simulink model "Regularization"  (Simulink 7.6)
settings: Solver=FixedStepDiscrete  StartTime=0.0  StopTime=60*60*4  FixedStep=300  RelTol=1e-3
values from neighbouring files (symbols this model uses):
  A_ahuflow = [1 0]    [RegularizationData.mat]
  A_DATtoZones = [1 0 0 0 0 0 0 0 0 0 0 0 ... (648 elements, 18x36)]    [RegularizationData.mat]
  A_fan_sup = [3 2 1 0]    [RegularizationData.mat]
  A_mapMatrixVAV2Zones1 = [1 0 0 0 0 0 0 0 0 0 0 0 ... (324 elements, 18x18)]    [RegularizationData.mat]
  A_mdots_boundsMax = [1 0 0 0 0 0 0 0 0 0 0 0 ... (1296 elements, 36x36)]    [RegularizationData.mat]
  A_mdots_boundsMin = [1 0 0 0 0 0 0 0 0 0 0 0 ... (1296 elements, 36x36)]    [RegularizationData.mat]
  A_OADtoOAF = [2 1 0]    [RegularizationData.mat]
  A_ObjFun = [1 0 0 0 0 1 0 0 0 0 1 0 ... (20 elements, 4x5)]    [RegularizationData.mat]
  A_returnT1 = [1 0 0 0 0 0 0 0 0 0 0 0 ... (324 elements, 18x18)]    [RegularizationData.mat]
  A_sum_DAT = [1 0 0 0 0 0 0 0 0 0 0 0 ... (361 elements, 19x19)]    [RegularizationData.mat]
  A_sumMdots1 = [1 0 0 0 0 0 0 0 0 0 0 0 ... (324 elements, 18x18)]    [RegularizationData.mat]
  A_Tzone_bounds1 = [1 0 0 0 0 0 0 0 0 0 0 0 ... (729 elements, 27x27)]    [RegularizationData.mat]
  A_VAV_DAT = [1 1 1 1 1 1 1 1 1 1 1 1 ... (666 elements, 18x37)]    [RegularizationData.mat]
  A_VAV_Energy = [0 1 0 1 0 1 0 1 0 1 0 1 ... (1332 elements, 36x37)]    [RegularizationData.mat]
  A_vlvcomd_boundsMax = [1 0 0 0 0 0 0 0 0 0 0 0 ... (1296 elements, 36x36)]    [RegularizationData.mat]
  A_vlvcomd_boundsMin = [1 0 0 0 0 0 0 0 0 0 0 0 ... (1296 elements, 36x36)]    [RegularizationData.mat]
  Azone =     [RegularizationData.mat]
  C_ahuflow = [0.90501 7.4491]    [RegularizationData.mat]
  C_DATtoZones = [1 0 0 0 0 0 0 0 0 1 0 0 ... (162 elements, 9x18)]    [RegularizationData.mat]
  C_fan_sup = [0.007418 -0.1732 2.207 -5.847]    [RegularizationData.mat]
  C_mapMatrixVAV2Zones1 = [1 0 0 0 0 0 0 0 0 0.813953488 0 0 ... (162 elements, 9x18)]    [RegularizationData.mat]
  C_mdots_boundsMax = [1 0 0 0 0 0 0 0 0 0 0 0 ... (648 elements, 18x36)]    [RegularizationData.mat]
  C_mdots_boundsMin = [1 0 0 0 0 0 0 0 0 0 0 0 ... (648 elements, 18x36)]    [RegularizationData.mat]
  C_OADtoOAF = [-2.3694 4.3066 -1.008]    [RegularizationData.mat]
  C_ObjFun = [3 1 1 1]    [RegularizationData.mat]
  C_returnT1 = [1 1 1 1 1 1 1 1 1 -0.4 -0.4 -0.4 ... (18 elements, 1x18)]    [RegularizationData.mat]
  C_sum_DAT = [1 1 1 1 1 1 1 1 1 1 1 1 ... (342 elements, 18x19)]    [RegularizationData.mat]
  C_sumMdots1 = [1 1 1 1 1 1 1 1 1 1 1 1 ... (18 elements, 1x18)]    [RegularizationData.mat]
  C_Tzone_boundsMax1 = [1 0 0 0 0 0 0 0 0 0 1 0 ... (243 elements, 9x27)]    [RegularizationData.mat]
  C_Tzone_boundsMin1 = [1 0 0 0 0 0 0 0 0 0 1 0 ... (243 elements, 9x27)]    [RegularizationData.mat]
  C_VAV_DAT = [0.253505482147 0 0 0 0 0 0 0 0 0 0 0 ... (324 elements, 18x18)]    [RegularizationData.mat]
  C_VAV_Energy = [1 0 0 0 0 0 0 0 0 0 0 0 ... (648 elements, 18x36)]    [RegularizationData.mat]
  C_vlvcomd_boundsMax = [1 0 0 0 0 0 0 0 0 0 0 0 ... (648 elements, 18x36)]    [RegularizationData.mat]
  C_vlvcomd_boundsMin = [1 0 0 0 0 0 0 0 0 0 0 0 ... (648 elements, 18x36)]    [RegularizationData.mat]
  cp_air = 1.006    [RegularizationData.mat]
  cp_w = 4.18    [RegularizationData.mat]
  Czone =     [RegularizationData.mat]
  d = [0.040172538 0.168105054 0.715382539]    [RegularizationData.mat]
  DAT_init = 18.3333333333    [RegularizationData.mat]
  DAT_max_init = 24.4444444444    [RegularizationData.mat]
  DAT_min_init = 12.7777777778    [RegularizationData.mat]
  DAT_step_cost = 5    [RegularizationData.mat]
  dTfan_const = 1    [RegularizationData.mat]
  eff_hc_max = 0.7    [RegularizationData.mat]
  HWST_init = 48.8888888889    [RegularizationData.mat]
  MaxAirFlow1 = 22.6524    [RegularizationData.mat]
  MaxZoneT = [26 26 26 26 26 26 26 26 26]    [RegularizationData.mat]
  mdotsa_init = [0.25 0.25 0.25 0.25 0.25 0.25 0.25 0.25 0.25 0.25 0.25 0.25 ... (18 elements, 18x1)]    [RegularizationData.mat]
  mdotsa_vav_max = [2 2 2 2 2 2 2 2 2 2 2 2 ... (18 elements, 18x1)]    [RegularizationData.mat]
  mdotsa_vav_min = [0.2 0.2 0.2 0.2 0.2 0.2 0.2 0.2 0.2 0.2 0.2 0.2 ... (18 elements, 18x1)]    [RegularizationData.mat]
  mdotw_max = 5.868    [RegularizationData.mat]
  MinAirFlow1 = 2.03881295462    [RegularizationData.mat]
  MinZoneT = [19 19 19 19 19 19 19 19 19]    [RegularizationData.mat]
  NumVAV1 = 18    [RegularizationData.mat]
  NumZones1 = 9    [RegularizationData.mat]
  OAD_high = 1    [RegularizationData.mat]
  OAD_init = 0.5    [RegularizationData.mat]
  OAD_low = 0.3    [RegularizationData.mat]
  params =     [RegularizationData.mat]
  SlackVariable_Weight = 10000    [RegularizationData.mat]
  vlvcomd_init = [0.01 0.01 0.01 0.01 0.01 0.01 0.01 0.01 0.01 0.01 0.01 0.01 ... (18 elements, 1x18)]    [RegularizationData.mat]
  vlvcomd_vav_high = [1 1 1 1 1 1 1 1 1 1 1 1 ... (18 elements, 18x1)]    [RegularizationData.mat]
  vlvcomd_vav_low = [0.002 0.002 0.002 0.002 0.002 0.002 0.002 0.002 0.002 0.002 0.002 0.002 ... (18 elements, 18x1)]    [RegularizationData.mat]
  vlvComdMin = [0.001 0.001 0.001 0.001 0.001 0.001 0.001 0.001 0.001 0.001 0.001 0.001 ... (18 elements, 18x1)]    [RegularizationData.mat]
undefined symbols (not defined in the file or in its folder): DAT, DAT_min, DAT_min_ext, dTfan, MAT, mdot_a, mdotsa, mdotsa_SP, OAD, prevDAT, slack, slack_weight, sparse, T, Thd, Thws, TLB, Tmix, TUB, Twin, vav_energy, vlv, vlv_comd, x1, x2
libraries: MPCMdlLib x75
settings Model: Creator=trckam  LastModifiedBy=sergv

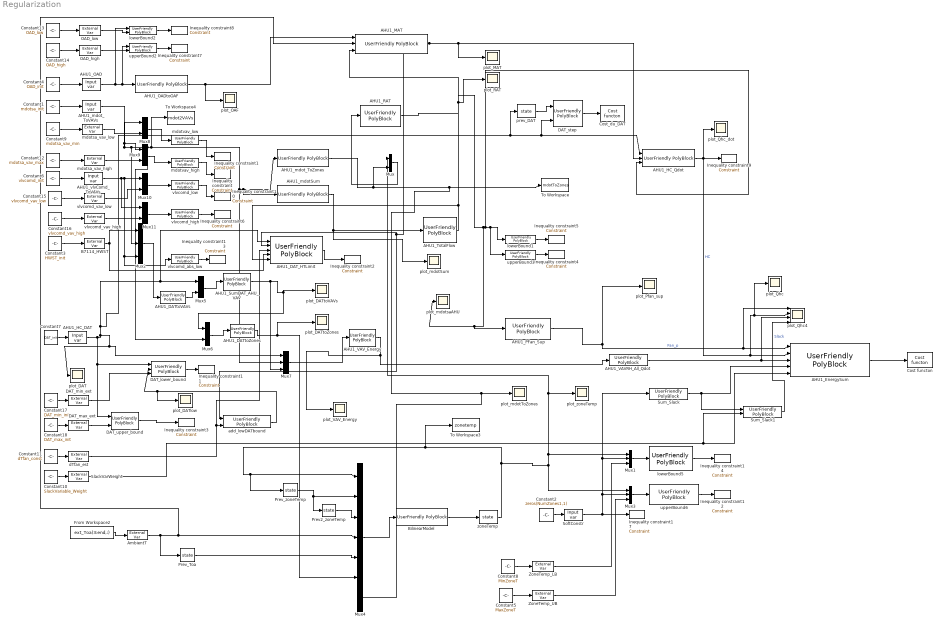
== system Regularization ==
  AHU1_DAT_HTLimit : MPCMdlLib/UserFriendly PolyBlock  Tag=PolyBlock  A=[1 0 0 0 1;0 1 0 0 1;0 0 1 0 1;0 1 0 0 0;0 0 0 1 0]  C=[cp_air, -cp_air, -cp_air, +eff_hc_max*mdotw_max*cp_w, -eff_hc_max*mdotw_max*cp_w]  gA=[0 0 0 0 0]  gC=[1]  input_type=Scalar  output_type=Scalar  port_names=DAT,MAT,dTfan,Twin,mdotsa
  AHU1_DATtoVAVs : MPCMdlLib/UserFriendly PolyBlock  Tag=PolyBlock  A=A_VAV_DAT  C=C_VAV_DAT  gA=zeros(1,37)  gC=[1]  input_type=Vector  output_type=Vector  port_names=Thws,mdotsa_SP[1-18],vlv_comd[1-18]
  AHU1_DATtoZones : MPCMdlLib/UserFriendly PolyBlock  Tag=PolyBlock  A=A_DATtoZones  C=C_DATtoZones  gA=Ag_DATtoZones  gC=Cg_DATtoZones  input_type=Vector  output_type=Vector  port_names=x1,x2
  AHU1_EnergySum : MPCMdlLib/UserFriendly PolyBlock  Tag=PolyBlock  A=A_ObjFun  C=C_ObjFun  gA=zeros(1,size(A_ObjFun,2))  gC=1  input_type=Scalar  output_type=Scalar  port_names=Pfan, Qhc, Qrh,slack,slack_weight
  AHU1_HC_DAT : MPCMdlLib/Input var  Tag=OptInput  SystemSampleTime=-1  step_ratio=1  save_name=BL_AHU1_HC_DAT
  AHU1_HC_Qdot : MPCMdlLib/UserFriendly PolyBlock  Tag=PolyBlock  A=[1 0 1;0 1 1;0 0 1]  C=[cp_air, -cp_air, -cp_air]  gA=[0 0 0]  gC=[1]  input_type=Scalar  output_type=Scalar  port_names=Thd,Tmix,mdot_a
  AHU1_MAT : MPCMdlLib/UserFriendly PolyBlock  Tag=PolyBlock  A=[1 1 0; 0 0 1;1 0 1]  C=[1 1 -1]  gA=[0 0 0]  gC=1  input_type=Scalar  output_type=Scalar  port_names=frac,amb, ret
  AHU1_OAD : MPCMdlLib/Input var  Tag=OptInput  SystemSampleTime=-1  step_ratio=1  save_name=BL_AHU1_OAD
  AHU1_OADtoOAF : MPCMdlLib/UserFriendly PolyBlock  Tag=PolyBlock  A=A_OADtoOAF  C=C_OADtoOAF  gA=[0]  gC=1  input_type=Scalar  output_type=Scalar  port_names=OAD
  AHU1_PFan_Sup : MPCMdlLib/UserFriendly PolyBlock  Tag=PolyBlock  A=A_fan_sup  C=C_fan_sup  gA=[0 ]  gC=1  input_type=Scalar  output_type=Scalar  port_names=mdot_a
  AHU1_RAT : MPCMdlLib/UserFriendly PolyBlock  Tag=PolyBlock  A=A_returnT1  C=C_returnT1  gA=gA_returnT1  gC=Cg_returnT1  input_type=Vector  output_type=Scalar  port_names=x1,x2
  AHU1_SumDAT_AHU_VAV : MPCMdlLib/UserFriendly PolyBlock  Tag=PolyBlock  A=A_sum_DAT  C=C_sum_DAT  gA=zeros(1,19)  gC=1  input_type=Vector  output_type=Vector  port_names=x1,x2
  AHU1_TotalFlow : MPCMdlLib/UserFriendly PolyBlock  Tag=PolyBlock  A=A_ahuflow  C=C_ahuflow  gA=[ 0]  gC=1  input_type=Scalar  output_type=Scalar  port_names=mdotvav
  AHU1_VAVRH_All_Qdot : MPCMdlLib/UserFriendly PolyBlock  Tag=PolyBlock  A=eye(NumVAV1)  C=ones(1,NumVAV1)  gA=zeros(1,NumVAV1)  gC=1  input_type=Vector  output_type=Scalar  port_names=vav_energy[1-9]
  AHU1_VAV_Energy : MPCMdlLib/UserFriendly PolyBlock  Tag=PolyBlock  A=A_VAV_Energy  C=C_VAV_Energy  gA=zeros(1,37)  gC=1  input_type=Vector  output_type=Vector  port_names=x1,x2
  AHU1_mdotSum : MPCMdlLib/UserFriendly PolyBlock  Tag=PolyBlock  A=A_sumMdots1  C=C_sumMdots1  gA=sparse(1,size(A_sumMdots1,2),0)  gC=1  input_type=Vector  output_type=Vector  port_names=x1,x2
  AHU1_mdot_ToVAVs : MPCMdlLib/Input var  Tag=OptInput  SystemSampleTime=-1  step_ratio=1  save_name=BL_AHU1_mdot_ToVAVs
  AHU1_mdot_ToZones : MPCMdlLib/UserFriendly PolyBlock  Tag=PolyBlock  A=A_mapMatrixVAV2Zones1  C=C_mapMatrixVAV2Zones1  gA=sparse(1,size(A_mapMatrixVAV2Zones1,2),0)  gC=1  input_type=Vector  output_type=Vector  port_names=x1,x2
  AHU1_vlvComd_ToVAVs : MPCMdlLib/Input var  Tag=OptInput  SystemSampleTime=-1  step_ratio=1  save_name=BL_AHU1_vlvComd_ToVAVs
  AmbientT : MPCMdlLib/External Var  Tag=OptExternal  SystemSampleTime=-1  save_name=BL_AmbientT
  B7114_HWST : MPCMdlLib/External Var  Tag=OptExternal  SystemSampleTime=-1  save_name=BL_B7114_HWST
  BilinearModel : MPCMdlLib/UserFriendly PolyBlock  Tag=PolyBlock  A=Azone  C=Czone  gA=sparse(1,size(Azone,2),0)  gC=1  input_type=Vector  output_type=Vector  port_names=UU
  Constant1 : Constant  Value=mdotsa_init
  Constant10 : Constant  Value=SlackVariable_Weight
  Constant11 : Constant  Value=dTfan_const
  Constant12 : Constant  Value=mdotsa_vav_max
  Constant13 : Constant  Value=OAD_low
  Constant14 : Constant  Value=OAD_high
  Constant15 : Constant  Value=vlvcomd_vav_low
  Constant16 : Constant  Value=vlvcomd_vav_high
  Constant17 : Constant  Value=DAT_min_init
  Constant18 : Constant  Value=DAT_max_init
  Constant2 : Constant  Value=zeros(NumZones1,1)
  Constant3 : Constant  Value=HWST_init
  Constant4 : Constant  Value=OAD_init
  Constant5 : Constant  Value=MaxZoneT
  Constant6 : Constant  Value=vlvcomd_init
  Constant7 : Constant  Value=DAT_init
  Constant8 : Constant  Value=MinZoneT
  Constant9 : Constant  Value=mdotsa_vav_min
  Cost functon : MPCMdlLib/Cost functon  Tag=OptCost
  "Cost_du_DAT " : MPCMdlLib/Cost functon  Tag=OptCost
  DAT_lower_bound : MPCMdlLib/UserFriendly PolyBlock  Tag=PolyBlock  A=[1 0 0;0 1 0;0 0 1]  C=[1 -1 0;1 0 -1]  gA=[0 0 0]  gC=1  input_type=Scalar  output_type=Vector  port_names=DAT,DAT_min,DAT_min_ext
  DAT_max_ext : MPCMdlLib/External Var  Tag=OptExternal  SystemSampleTime=-1  save_name=BL_DAT_max_ext
  DAT_min_ext : MPCMdlLib/External Var  Tag=OptExternal  SystemSampleTime=-1  save_name=BL_DAT_min_ext
  DAT_step : MPCMdlLib/UserFriendly PolyBlock  Tag=PolyBlock  A=[2 0 ; 1 1 ; 0 2]  C=[1 -2 1]*DAT_step_cost  gA=[0 0]  gC=1  input_type=Scalar  output_type=Scalar  port_names=DAT,prevDAT
  DAT_upper_bound : MPCMdlLib/UserFriendly PolyBlock  Tag=PolyBlock  A=[1 0;0 1]  C=[1 -1]  gA=[0 0]  gC=1  input_type=Scalar  output_type=Scalar  port_names=DAT, DAT_max
  From Workspace2 : FromWorkspace  VariableName=ext_Toa(3:end,:)  SampleTime=300
  Inequality constraint{,2..4,6..7,12} (7 alike) : MPCMdlLib/Constraint  Tag=InequalBlock  CompareSign=< 0
  Inequality constraint{1,5,8..11,13..14,17} (9 alike) : MPCMdlLib/Constraint  Tag=InequalBlock  CompareSign=> 0
  Mux{,5..6,8..11} (7 alike) : Mux  Inputs=2
  Mux{1..3,7} (4 alike) : Mux  Inputs=3
  Mux4 : Mux  Inputs=7
  OAD_high : MPCMdlLib/External Var  Tag=OptExternal  SystemSampleTime=-1  save_name=BL_OAD_high
  OAD_low : MPCMdlLib/External Var  Tag=OptExternal  SystemSampleTime=-1  save_name=BL_OAD_low
  Prev2_zoneTemp : MPCMdlLib/state  Tag=OptState  SystemSampleTime=-1  init_val=params.y0(1,:)  save_name=BL_Prev2_zoneTemp
  Prev_Toa : MPCMdlLib/state  Tag=OptState  SystemSampleTime=-1  init_val=ext_Toa(2,2:end)  save_name=BL_Prev_Toa
  Prev_zoneTemp : MPCMdlLib/state  Tag=OptState  SystemSampleTime=-1  init_val=params.y0(2,:)  save_name=BL_Prev_zoneTemp
  SlackVarWeight : MPCMdlLib/External Var  Tag=OptExternal  SystemSampleTime=-1  save_name=BL_SlackVarWeight
  SoftConstr : MPCMdlLib/Input var  Tag=OptInput  SystemSampleTime=-1  step_ratio=1  save_name=BL_SoftConstr
  Sum_Slack : MPCMdlLib/UserFriendly PolyBlock  Tag=PolyBlock  A=eye(NumZones1)  C=ones(1,NumZones1)  gA=zeros(1,NumZones1)  gC=1  input_type=Vector  output_type=Scalar  port_names=slack[1-1000]
  Sum_Slack1 : MPCMdlLib/UserFriendly PolyBlock  Tag=PolyBlock  A=[1 1]  C=[1]  gA=[0 0]  gC=1  input_type=Scalar  output_type=Scalar  port_names=slack,slack_weight
  To Workspace : ToWorkspace  VariableName=mdotToZones  SampleTime=-1  SaveFormat=Structure
  To Workspace3 : ToWorkspace  VariableName=zonetemp  SampleTime=-1  SaveFormat=Structure
  To Workspace4 : ToWorkspace  VariableName=mdot2VAVs  SampleTime=-1  SaveFormat=Structure
  ZoneTemp_LB : MPCMdlLib/External Var  Tag=OptExternal  SystemSampleTime=-1  save_name=BL_ZoneTemp_LB
  ZoneTemp_UB : MPCMdlLib/External Var  Tag=OptExternal  SystemSampleTime=-1  save_name=BL_ZoneTemp_UB
  add_lowDATbound : MPCMdlLib/UserFriendly PolyBlock  Tag=PolyBlock  A=[1 0;0 1]  C=[1 1]  gA=[0 0]  gC=1  input_type=Scalar  output_type=Scalar  port_names=MAT,dTfan
  dTfan_est : MPCMdlLib/External Var  Tag=OptExternal  SystemSampleTime=-1  save_name=BL_dTfan_est
  lowerBound1 : MPCMdlLib/UserFriendly PolyBlock  Tag=PolyBlock  A=[1; 0]  C=[1 -MinAirFlow1]  gA=[0 ]  gC=1  input_type=Scalar  output_type=Scalar  port_names=x1
  lowerBound2 : MPCMdlLib/UserFriendly PolyBlock  Tag=PolyBlock  A=[1 0;0 1]  C=[1 -1]  gA=[0 0]  gC=1  input_type=Scalar  output_type=Scalar  port_names=OAD, OAD_low
  lowerBound5 : MPCMdlLib/UserFriendly PolyBlock  Tag=PolyBlock  A=A_Tzone_bounds1  C=C_Tzone_boundsMin1  gA=sparse(1,size(A_Tzone_bounds1,2),0)  gC=1  input_type=Vector  output_type=Vector  port_names=T[1-9],d[1-9],TLB[1-9]
  mdotsa_vav_high : MPCMdlLib/External Var  Tag=OptExternal  SystemSampleTime=-1  save_name=BL_mdotsa_vav_high
  mdotsa_vav_low : MPCMdlLib/External Var  Tag=OptExternal  SystemSampleTime=-1  save_name=BL_mdotsa_vav_low
  mdotvav_high : MPCMdlLib/UserFriendly PolyBlock  Tag=PolyBlock  A=A_mdots_boundsMax  C=C_mdots_boundsMax  gA=sparse(1,size(A_mdots_boundsMax,2),0)  gC=1  input_type=Vector  output_type=Vector  port_names=x1,x2
  mdotvav_low : MPCMdlLib/UserFriendly PolyBlock  Tag=PolyBlock  A=A_mdots_boundsMin  C=C_mdots_boundsMin  gA=sparse(1,size(A_mdots_boundsMin,2),0)  gC=1  input_type=Vector  output_type=Vector  port_names=x1,x2
  plot_DAT : Scope
      settings: TimeRange=6000  YMin=21.30200235571261  YMax=22.1020023557126  SaveName=ScopeData11
  plot_DATlow : Scope
      settings: TimeRange=6000  YMin=21.30200235571261  YMax=22.1020023557126  SaveName=ScopeData12
  plot_DATtoVAVs : Scope
      settings: TimeRange=6000  YMin=21.30200235571261  YMax=22.1020023557126
  plot_DATtoZones : Scope
      settings: TimeRange=6000  YMin=21.30200235571261  YMax=22.1020023557126  SaveName=ScopeData3
  plot_MAT : Scope
      settings: TimeRange=15000  YMin=20  YMax=25  SaveName=ScopeData10
  plot_OAF : Scope
      settings: TimeRange=14400  YMin=21.25  YMax=24.5  SaveName=ScopeData7
  plot_Pfan_sup : Scope
      settings: TimeRange=14400  YMin=21.25  YMax=24.5  SaveName=ScopeData2
  plot_Qhc : Scope
      settings: TimeRange=14400  YMin=21.25  YMax=24.5  SaveName=ScopeData13
  plot_Qhc4 : Scope  NumInputPorts=4
      settings: TimeRange=14400  YMin=21.25~-5~-5~-5  YMax=24.5~5~5~5  SaveName=ScopeData17
  plot_Qhc_dot : Scope
      settings: TimeRange=15000  YMin=89  YMax=96  SaveName=ScopeData6
  plot_RAT : Scope
      settings: TimeRange=14400  YMin=9.236459999999999  YMax=10.2087  SaveName=ScopeData5
  plot_VAV_Energy : Scope
      settings: TimeRange=6000  YMin=8  YMax=24  SaveName=ScopeData9
  plot_mdotSum : Scope
      settings: YMin=9.23646  YMax=10.2087  SaveName=ScopeData4
  plot_mdotToZones : Scope
      settings: TimeRange=14400
  plot_mdotsaAHU : Scope
      settings: TimeRange=14400  YMin=21.25  YMax=24.5  SaveName=ScopeData8
  plot_zoneTemp : Scope
      settings: YMin=21.25  YMax=24.5  SaveName=ScopeData15
  prev_DAT : MPCMdlLib/state  Tag=OptState  SystemSampleTime=-1  init_val=20  save_name=BL_prev_DAT
  upperBound2 : MPCMdlLib/UserFriendly PolyBlock  Tag=PolyBlock  A=[1 0;0 1]  C=[1 -1]  gA=[0 0]  gC=1  input_type=Scalar  output_type=Scalar  port_names=OAD,OAD_high
  upperBound3 : MPCMdlLib/UserFriendly PolyBlock  Tag=PolyBlock  A=[1;0]  C=[1 -MaxAirFlow1]  gA=[0]  gC=1  input_type=Scalar  output_type=Scalar  port_names=x1,x2
  upperBound6 : MPCMdlLib/UserFriendly PolyBlock  Tag=PolyBlock  A=A_Tzone_bounds1  C=C_Tzone_boundsMax1  gA=sparse(1,size(A_Tzone_bounds1,2),0)  gC=1  input_type=Vector  output_type=Vector  port_names=T[1-9],d[1-9],TUB[1-9]
  vlvcomd_abs_low : MPCMdlLib/UserFriendly PolyBlock  Tag=PolyBlock  A=[eye(NumVAV1); zeros(1,NumVAV1)]  C="[eye(NumVAV1)  -vlvComdMin(1:NumVAV1)]"  gA=sparse(1,NumVAV1,0)  gC=1  input_type=Vector  output_type=Vector  port_names=vlv[1-18]
  vlvcomd_high : MPCMdlLib/UserFriendly PolyBlock  Tag=PolyBlock  A=A_vlvcomd_boundsMax  C=C_vlvcomd_boundsMax  gA=sparse(1,size(A_vlvcomd_boundsMax,2),0)  gC=1  input_type=Vector  output_type=Vector  port_names=x1,x2
  vlvcomd_low : MPCMdlLib/UserFriendly PolyBlock  Tag=PolyBlock  A=A_vlvcomd_boundsMin  C=C_vlvcomd_boundsMin  gA=sparse(1,size(A_vlvcomd_boundsMin,2),0)  gC=1  input_type=Vector  output_type=Vector  port_names=x1,x2
  vlvcomd_vav_high : MPCMdlLib/External Var  Tag=OptExternal  SystemSampleTime=-1  save_name=BL_vlvcomd_vav_high
  vlvcomd_vav_low : MPCMdlLib/External Var  Tag=OptExternal  SystemSampleTime=-1  save_name=BL_vlvcomd_vav_low
  zoneTemp : MPCMdlLib/state  Tag=OptState  SystemSampleTime=-1  init_val=params.y0(3,:)  save_name=BL_zoneTemp
  wires:
  Constant1/1 -> AHU1_mdot_ToVAVs/1
  AHU1_mdot_ToVAVs/1 -> Mux9/1, Mux8/1, Mux2/2, To Workspace4/1, AHU1_mdot_ToZones/1, AHU1_mdotSum/1, Mux7/2, Mux6/2
  Mux/1 -> AHU1_RAT/1
  mdotvav_high/1 -> Inequality constraint/1
  mdotvav_low/1 -> Inequality constraint1/1
  upperBound3/1 -> Inequality constraint4/1
  lowerBound1/1 -> Inequality constraint5/1
  AHU1_mdot_ToZones/1 -> To Workspace/1, plot_mdotToZones/1, Mux4/7, Mux/2
  AHU1_EnergySum/1 -> Cost functon/1
  Constant7/1 -> AHU1_HC_DAT/1
  AHU1_HC_DAT/1 -> DAT_upper_bound/1, DAT_lower_bound/1, Mux5/1, AHU1_DAT_HTLimit/1, prev_DAT/1, AHU1_HC_Qdot/1, DAT_step/2, Mux7/1, plot_DAT/1
  upperBound6/1 -> Inequality constraint12/1
  lowerBound5/1 -> Inequality constraint14/1
  Constant2/1 -> SoftConstr/1
  SoftConstr/1 -> Mux3/2, Sum_Slack/1, Mux1/2, Inequality constraint17/1
  Mux1/1 -> lowerBound5/1
  Mux3/1 -> upperBound6/1
  BilinearModel/1 -> zoneTemp/1
  zoneTemp/1 -> Mux4/1, Prev_zoneTemp/1, To Workspace3/1, plot_zoneTemp/1, Mux/1, Mux1/1, Mux3/1
  Prev_zoneTemp/1 -> Mux4/2, Prev2_zoneTemp/1
  AmbientT/1 -> Prev_Toa/1, Mux4/4, AHU1_MAT/2
  From Workspace2/1 -> AmbientT/1
  Mux4/1 -> BilinearModel/1
  Prev2_zoneTemp/1 -> Mux4/3
  Constant5/1 -> ZoneTemp_UB/1
  Constant8/1 -> ZoneTemp_LB/1
  ZoneTemp_LB/1 -> Mux1/3
  ZoneTemp_UB/1 -> Mux3/3
  Constant10/1 -> SlackVarWeight/1
  Prev_Toa/1 -> Mux4/5
  AHU1_mdotSum/1 -> plot_mdotSum/1, AHU1_TotalFlow/1
  AHU1_TotalFlow/1 -> AHU1_PFan_Sup/1, plot_mdotsaAHU/1, upperBound3/1, lowerBound1/1, AHU1_HC_Qdot/3, AHU1_DAT_HTLimit/5
  AHU1_OAD/1 -> AHU1_OADtoOAF/1, upperBound2/1, lowerBound2/1
  Constant4/1 -> AHU1_OAD/1
  lowerBound2/1 -> Inequality constraint8/1
  upperBound2/1 -> Inequality constraint7/1
  AHU1_PFan_Sup/1 -> plot_Qhc4/1, AHU1_EnergySum/1, plot_Pfan_sup/1  "Fan_p"
  AHU1_OADtoOAF/1 -> AHU1_MAT/1, plot_OAF/1
  AHU1_HC_Qdot/1 -> plot_Qhc4/2, plot_Qhc/1, AHU1_EnergySum/2, Inequality constraint9/1, plot_Qhc_dot/1  "HC"
  AHU1_MAT/1 -> plot_MAT/1, AHU1_HC_Qdot/2, add_lowDATbound/1, AHU1_DAT_HTLimit/2
  Constant3/1 -> B7114_HWST/1
  Constant6/1 -> AHU1_vlvComd_ToVAVs/1
  AHU1_vlvComd_ToVAVs/1 -> Mux10/1, Mux2/3, vlvcomd_abs_low/1, Mux11/1
  B7114_HWST/1 -> Mux2/1, AHU1_DAT_HTLimit/4
  Mux2/1 -> AHU1_DATtoVAVs/1
  AHU1_DATtoVAVs/1 -> Mux5/2
  Mux5/1 -> AHU1_SumDAT_AHU_VAV/1
  AHU1_SumDAT_AHU_VAV/1 -> plot_DATtoVAVs/1, Mux6/1, Mux7/3
  AHU1_DATtoZones/1 -> Mux4/6, plot_DATtoZones/1
  Mux6/1 -> AHU1_DATtoZones/1
  vlvcomd_low/1 -> Inequality constraint10/1
  vlvcomd_high/1 -> Inequality constraint6/1
  Mux7/1 -> AHU1_VAV_Energy/1
  AHU1_VAV_Energy/1 -> plot_VAV_Energy/1, AHU1_VAVRH_All_Qdot/1
  AHU1_RAT/1 -> plot_RAT/1, AHU1_MAT/3
  SlackVarWeight/1 -> Sum_Slack1/2, AHU1_EnergySum/5
  Sum_Slack/1 -> Sum_Slack1/1, AHU1_EnergySum/4
  AHU1_VAVRH_All_Qdot/1 -> plot_Qhc4/3, AHU1_EnergySum/3
  Sum_Slack1/1 -> plot_Qhc4/4  "Slack"
  Mux8/1 -> mdotvav_low/1
  Constant9/1 -> mdotsa_vav_low/1
  mdotsa_vav_low/1 -> Mux8/2
  Constant11/1 -> dTfan_est/1
  dTfan_est/1 -> AHU1_DAT_HTLimit/3, add_lowDATbound/2
  add_lowDATbound/1 -> plot_DATlow/1, DAT_lower_bound/2
  DAT_lower_bound/1 -> Inequality constraint11/1
  DAT_upper_bound/1 -> Inequality constraint3/1
  AHU1_DAT_HTLimit/1 -> Inequality constraint2/1
  Constant12/1 -> mdotsa_vav_high/1
  mdotsa_vav_high/1 -> Mux9/2
  Mux9/1 -> mdotvav_high/1
  Constant13/1 -> OAD_low/1
  Constant14/1 -> OAD_high/1
  OAD_low/1 -> lowerBound2/2
  OAD_high/1 -> upperBound2/2
  Mux10/1 -> vlvcomd_low/1
  vlvcomd_vav_low/1 -> Mux10/2
  Constant15/1 -> vlvcomd_vav_low/1
  Mux11/1 -> vlvcomd_high/1
  vlvcomd_vav_high/1 -> Mux11/2
  Constant16/1 -> vlvcomd_vav_high/1
  vlvcomd_abs_low/1 -> Inequality constraint13/1
  prev_DAT/1 -> DAT_step/1
  DAT_min_ext/1 -> DAT_lower_bound/3
  Constant17/1 -> DAT_min_ext/1
  Constant18/1 -> DAT_max_ext/1
  DAT_max_ext/1 -> DAT_upper_bound/2
  DAT_step/1 -> "Cost_du_DAT "/1
